simulink model "WP_tippinig"  (R2023b)
settings: Solver=VariableStepAuto  StartTime=0.0  StopTime=40  RelTol=1e-3
settings Model: Creator=91996  LastModifiedBy=Dell

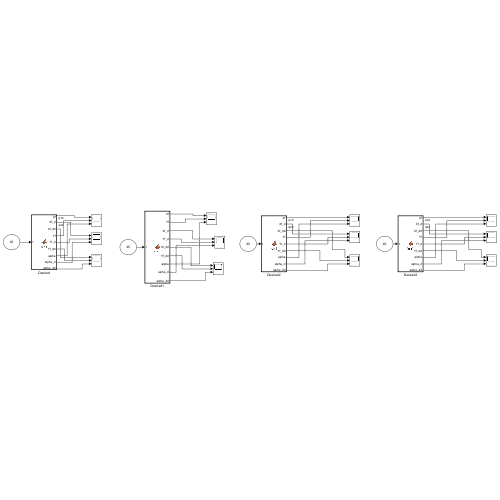
[thumbnail: Simulink's stored preview of the top-level diagram]
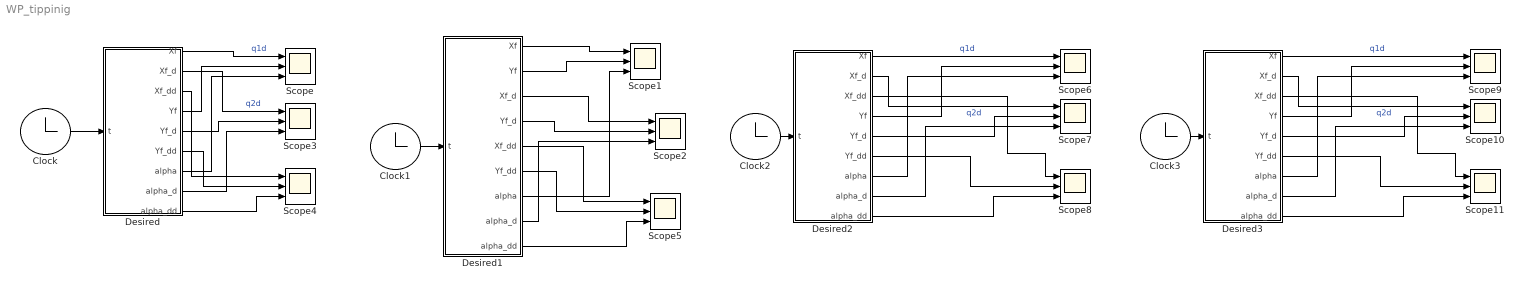
== system WP_tippinig ==
  Clock{,1..3} (4 alike) : Clock
  Desired : MATLAB Function  TreatAsAtomicUnit=on
  Desired1 : MATLAB Function  TreatAsAtomicUnit=on
  Desired2 : MATLAB Function  TreatAsAtomicUnit=on
  Desired3 : MATLAB Function  TreatAsAtomicUnit=on
  Scope{,1..11} (12 alike) : Scope  NumInputPorts=3
  wires:
  Clock/1 -> Desired/1(t)
  Desired/1(Xf) -> Scope/1  "q1d"
  Desired/2(Xf_d) -> Scope3/1  "q2d"
  Clock1/1 -> Desired1/1("t ")
  Desired1/3(Xf_d) -> Scope2/1
  Desired1/4(Yf_d) -> Scope2/2
  Desired1/5(Xf_dd) -> Scope5/1
  Desired1/6(Yf_dd) -> Scope5/2
  Desired1/7(alpha) -> Scope1/3
  Desired1/8(alpha_d) -> Scope2/3
  Desired1/9(alpha_dd) -> Scope5/3
  Desired1/1(Xf) -> Scope1/1
  Desired1/2(Yf) -> Scope1/2
  Desired/5(Yf_d) -> Scope3/2
  Desired/3(Xf_dd) -> Scope4/1
  Desired2/3(Xf_dd) -> Scope8/1
  Desired2/2(Xf_d) -> Scope7/1  "q2d"
  Clock2/1 -> Desired2/1(t)
  Desired/4(Yf) -> Scope/2
  Desired/6(Yf_dd) -> Scope4/2
  Desired/7(alpha) -> Scope/3
  Desired/8(alpha_d) -> Scope3/3
  Desired/9(alpha_dd) -> Scope4/3
  Desired2/1(Xf) -> Scope6/1  "q1d"
  Desired2/4(Yf) -> Scope6/2
  Desired2/5(Yf_d) -> Scope7/2
  Desired2/6(Yf_dd) -> Scope8/2
  Desired2/7(alpha) -> Scope6/3
  Desired2/8(alpha_d) -> Scope7/3
  Desired2/9(alpha_dd) -> Scope8/3
  Desired3/6(Yf_dd) -> Scope11/2
  Desired3/3(Xf_dd) -> Scope11/1
  Desired3/1(Xf) -> Scope9/1  "q1d"
  Desired3/8(alpha_d) -> Scope10/3
  Desired3/9(alpha_dd) -> Scope11/3
  Clock3/1 -> Desired3/1(t)
  Desired3/7(alpha) -> Scope9/3
  Desired3/5(Yf_d) -> Scope10/2
  Desired3/2(Xf_d) -> Scope10/1  "q2d"
  Desired3/4(Yf) -> Scope9/2

== matlab function WP_tippinig/Desired ==
  data: Xf output; Xf_d output; t input; Xf_dd output; Yf output; Yf_d output; Yf_dd output; alpha output; alpha_d output; alpha_dd output
function [Xf,Xf_d,Xf_dd,Yf,Yf_d,Yf_dd,alpha,alpha_d,alpha_dd]=fun1(t)
Xf0=0.65;
Xf0_d=0;
Xf0_dd=0;
Xfs=0.8;
Yfs=0.2;
ts=40;
[Xf,Xf_d,Xf_dd]=para_(Xf0,Xf0_d,Xf0_dd,t,ts,Xfs);
Yf=0.2;
Yf_d=0;
Yf_dd=0;
alpha=0;
alpha_d=0
alpha_dd=0;

== matlab function WP_tippinig/Desired2 ==
  data: Xf output; Xf_d output; t input; Xf_dd output; Yf output; Yf_d output; Yf_dd output; alpha output; alpha_d output; alpha_dd output
function [Xf,Xf_d,Xf_dd,Yf,Yf_d,Yf_dd,alpha,alpha_d,alpha_dd]=fun1(t)
Xf=0.8;
Xf_d=0;
Xf_dd=0;
Yf=0.2;
Yf_d=0;
Yf_dd=0;
ts=40;
alpha0=0.3;
alpha0_d=0;
alpha0_dd=0;
alphas=0;
[alpha,alpha_d,alpha_dd]=para_(alpha0,alpha0_d,alpha0_dd,t,ts,alphas);

== matlab function WP_tippinig/Desired3 ==
  data: Xf output; Xf_d output; t input; Xf_dd output; Yf output; Yf_d output; Yf_dd output; alpha output; alpha_d output; alpha_dd output
function [Xf,Xf_d,Xf_dd,Yf,Yf_d,Yf_dd,alpha,alpha_d,alpha_dd]=fun1(t)
Xf0=0.8;
Xf0_d=0;
Xf0_dd=0;
Xfs=0.9;
ts=40;
[Xf,Xf_d,Xf_dd]=para_(Xf0,Xf0_d,Xf0_dd,t,ts,Xfs);
Yf=0.2;
Yf_d=0;
Yf_dd=0;
alpha=0;
alpha_d=0
alpha_dd=0;

== matlab function WP_tippinig/Desired1 ==
  data: Xf output; Yf output; t input; Xf_d output; Yf_d output; Xf_dd output; Yf_dd output; alpha output; alpha_d output; alpha_dd output
function [Xf,Yf,Xf_d,Yf_d,Xf_dd,Yf_dd,alpha,alpha_d,alpha_dd]=fun1(t)
Xf=0.8;
Yf=0.2;
Xf_d=0;Xf_dd=0;
Yf_d=0;Yf_dd=0;
ts=40;
alpha0=0;
alpha0_d=0;
alpha0_dd=0;
alphas=0.3;
[alpha,alpha_d,alpha_dd]=para_(alpha0,alpha0_d,alpha0_dd,t,ts,alphas);
